simulink model "ball"  (R2020b)
settings: Solver=VariableStepAuto  StartTime=0.0  StopTime=10.0  RelTol=1e-3
settings Model: Creator=User  LastModifiedBy=User

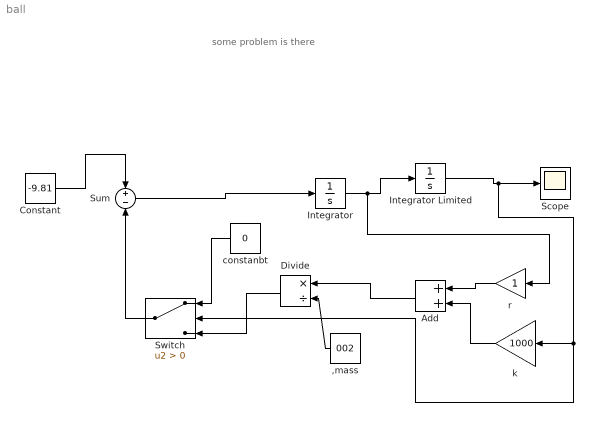
== system ball ==
  note: some problem is there
  ,mass : Constant  Value=002
  Add : Sum
  Constant : Constant  Value=-9.81
  Divide : Product  Inputs=*/
  Integrator : Integrator
  Integrator Limited : Integrator  LimitOutput=on  UpperSaturationLimit=1  LowerSaturationLimit=0
  Scope : Scope
  Sum : Sum  Inputs=+-
  Switch : Switch  Criteria=u2 > Threshold
  constanbt : Constant  Value=0
  k : Gain  Gain=1000
  r : Gain
  wires:
  Constant/1 -> Sum/1
  Sum/1 -> Integrator/1
  Integrator/1 -> r/1, Integrator Limited/1
  Integrator Limited/1 -> Switch/2, k/1, Scope/1
  r/1 -> Add/1
  k/1 -> Add/2
  ,mass/1 -> Divide/2
  Add/1 -> Divide/1
  constanbt/1 -> Switch/1
  Divide/1 -> Switch/3
  Switch/1 -> Sum/2
